simulink model "myMotor"  (R2023a)
settings: Solver=FixedStepAuto  StartTime=0.0  StopTime=10  FixedStep=0.005  RelTol=1e-3
undefined symbols (not defined in the file or in its folder): B_m, J_m, K_m, L_m, R_m
settings Model: Creator=sabir  LastModifiedBy=sabir
settings SolverCC: AlgebraicLoopSolver=TrustRegion
settings DebuggingCC: UnconnectedInputMsg=warning  UnconnectedOutputMsg=warning  UnconnectedLineMsg=warning
settings ModelReferenceCC: EnableRefExpFcnMdlSchedulingChecks=on

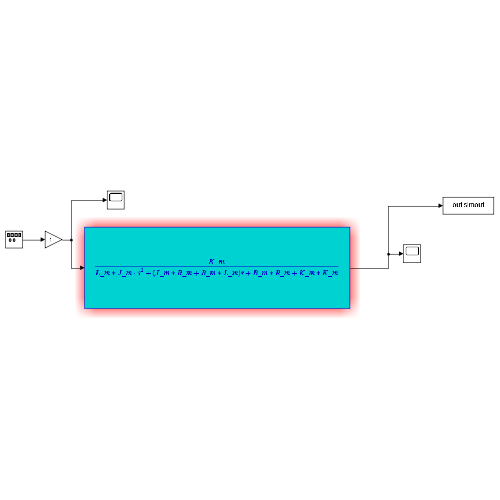
[thumbnail: Simulink's stored preview of the top-level diagram]
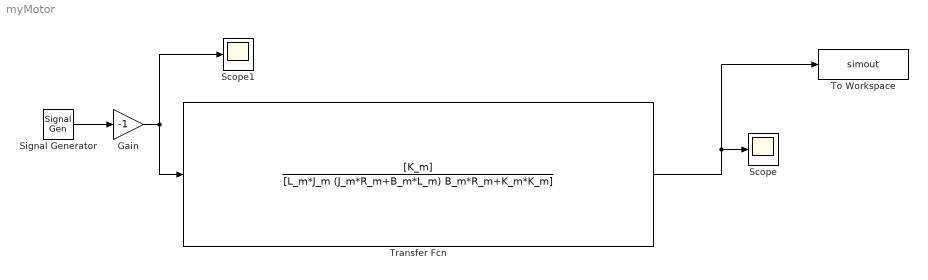
== system myMotor ==
  Gain : Gain  Gain=-1
  Scope : Scope
  Scope1 : Scope
  Signal Generator : SignalGenerator  WaveForm=square  Amplitude=12  Frequency=0.5
  To Workspace : ToWorkspace  VariableName=simout  SampleTime=-1
  Transfer Fcn : TransferFcn  Numerator=[K_m]  Denominator=[L_m*J_m (J_m*R_m+B_m*L_m) B_m*R_m+K_m*K_m]
  wires:
  Signal Generator/1 -> Gain/1
  Gain/1 -> Scope1/1, Transfer Fcn/1
  Transfer Fcn/1 -> To Workspace/1, Scope/1
